simulink model "modelo_identificacion"  (R2019b)
settings: Solver=VariableStepDiscrete  StartTime=0.0  StopTime=30.0  RelTol=1e-3
values from neighbouring files (symbols this model uses):
  Ts = 100e-3    (= 0.1)    [RunNARXposition.m]    (also in SimData.m)
settings Model: Creator=pizarro  LastModifiedBy=Laura
settings SFSimCC: CustomCodeUndefinedFunction=UseInterfaceOnly

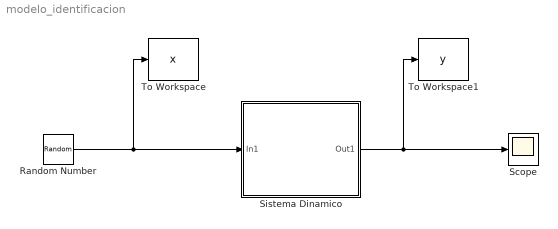
== system modelo_identificacion ==
  Random Number : RandomNumber  SampleTime=Ts
  Scope : Scope
  Sistema Dinamico : Subsystem
  To Workspace : ToWorkspace  VariableName=x  SaveFormat=Structure With Time  SampleTime=-1
      settings: Save2DSignal=2-D array (concatenate along first dimension)
  To Workspace1 : ToWorkspace  VariableName=y  SaveFormat=Structure With Time  SampleTime=-1
      settings: Save2DSignal=2-D array (concatenate along first dimension)
  wires:
  Random Number/1 -> To Workspace/1, Sistema Dinamico/1(In1)
  Sistema Dinamico/1(Out1) -> Scope/1, To Workspace1/1

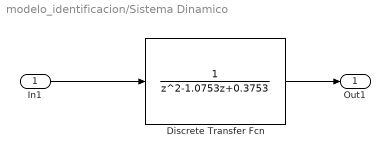
== system modelo_identificacion/Sistema Dinamico ==
  In1 : Inport
  Discrete Transfer Fcn : DiscreteTransferFcn  Denominator="[1.0000   -1.0753    0.3753]"  SampleTime=Ts
  Out1 : Outport  VectorParamsAs1DForOutWhenUnconnected=off
  wires:
  Discrete Transfer Fcn/1 -> Out1/1
  In1/1 -> Discrete Transfer Fcn/1
